simulink model "ScriptDemo"  (R2022b)
settings: configuration reference "TmVcThermal_Configuration_sub" (kept outside this file)
undefined symbols (not defined in the file or in its folder): aaaa, bbbb, cTmComprCtrl_D_u8HvacFlowTable_db, cTmComprCtrl_D_u8HvacFlowTable_sw, cTmComprCtrl_n_i16ChillCmpIMax, cTmComprCtrl_n_i16ChillCmpIMin, cTmComprCtrl_n_i16ChillCmpIMin666, cTmComprCtrl_n_i16ChillCmpPMax, cTmComprCtrl_n_i16ChillCmpPMin, cTmComprCtrl_n_i16CmpChillCoolRpmKiMax, cTmComprCtrl_n_i16CmpChillCoolRpmKiMin, cTmComprCtrl_n_i16CmpChillCoolRpmKpMax, cTmComprCtrl_n_i16CmpChillCoolRpmKpMin, cTmComprCtrl_n_i16CmpCoolRpmKiMax, cTmComprCtrl_n_i16CmpCoolRpmKiMin, cTmComprCtrl_n_i16CmpCoolRpmKpMax, cTmComprCtrl_n_i16CmpCoolRpmKpMin, cTmComprCtrl_n_i16SM4CmpHeatKiMax, cTmComprCtrl_n_i16SM4CmpHeatKiMin, cTmComprCtrl_n_i16SM4CmpHeatKpMax, cTmComprCtrl_n_i16SM4CmpHeatKpMin, cTmComprCtrl_n_i16SM5CmpHeatKiMax, cTmComprCtrl_n_i16SM5CmpHeatKiMin, cTmComprCtrl_n_i16SM5CmpHeatKpMax, cTmComprCtrl_n_i16SM5CmpHeatKpMin, cTmComprCtrl_n_i16SM6CmpHeatKiMax, cTmComprCtrl_n_i16SM6CmpHeatKiMin, cTmComprCtrl_n_i16SM6CmpHeatKpMax, cTmComprCtrl_n_i16SM6CmpHeatKpMin, cTmComprCtrl_n_u16CmpMaxSpdFanFltLimt, cTmComprCtrl_n_u16CmpMaxSpdLoSidePFltLimt, cTmComprCtrl_n_u16CmpMaxSpdSensorFltLimt, cTmComprCtrl_n_u16CompMinRpm, cTmComprCtrl_n_u16CompRpmIncThres, cTmComprCtrl_t_u16BattCooltFFPeriod, cTmComprCtrl_t_u16BattCooltPIPeriod, cTmComprCtrl_t_u16CmpCoolFFPeriod, cTmComprCtrl_t_u16CmpCoolPIPeriod, cTmComprCtrl_t_u16CoolCmpChillFFPeriod, cTmComprCtrl_t_u16CoolCmpChillPIPeriod, cTmComprCtrl_t_u16SM4CmpHeatFFPeriod, cTmComprCtrl_t_u16SM4CmpHeatPIPeriod, cTmComprCtrl_t_u16SM5CmpHeatFFPeriod, cTmComprCtrl_t_u16SM5CmpHeatPIPeriod, cTmComprCtrl_t_u16SM6CmpHeatFFPeriod, cTmComprCtrl_t_u16SM6CmpHeatPIPeriod, cTmComprCtrl_Te_EvapClearInteg, cTmComprCtrl_Te_i16HpReqTempSaturoffset, cTmComprCtrl_Te_i16SatLpReplaceDiff, cTmComprCtrl_Te_i16SM3BatDiffStartEvapDecOffset, cTmComprCtrl_Te_i16SM3EvapLo, cTmComprCtrl_Te_i16SM3TBatDiffEntEvapDecOffset, cTmComprCtrl_Te_i16SM3TBatDiffEntEvapDecOffsetQuit, cTmComprCtrl_Te_s32ErrCmpChillPIContinueCoolH, cTmComprCtrl_Te_s32ErrCmpChillPIContinueCoolL, cTmComprCtrl_Te_s32ErrCmpPIContinueChillH, cTmComprCtrl_Te_s32ErrCmpPIContinueChillL, cTmComprCtrl_Te_s32ErrCmpPIContinueCoolH, cTmComprCtrl_Te_s32ErrCmpPIContinueCoolL, cTmComprCtrl_Te_s32ErrCmpPIContinueHeatH ... (+398)
libraries: simulink x846, PCMULib x711, simulink_need_slupdate x4
(part 17 of 49)

== system ScriptDemo/Create/Model/createMode/Before ==
  note: % 目的: 为输出端口创建debug 及对应的输入模块
      | [cnt] = createDebug(gcs)
  sTmRefriVlvCtrl_X_s32CEXVPosReqIn : Inport  OutDataTypeStr=single
  sTmRefriVlvCtrl_X_s32EEXVPosReqIn : Inport  Port=2  OutDataTypeStr=single
  sTmRefriVlvCtrl_X_s32BEXVPosReqIn : Inport  Port=3  OutDataTypeStr=single
  yTmRefriVlvCtrl_B_HpcCexvMovEnableIn : Inport  Port=4  OutDataTypeStr=boolean
  sTmRefriVlvCtrl_Z_u8CEXVInitStateIn : Inport  Port=5  OutDataTypeStr=uint8
  yTmRefriVlvCtrl_B_CexvCalibReqIn : Inport  Port=6  OutDataTypeStr=boolean
  yTmRefriVlvCtrl_B_HpcEexvMovEnableIn : Inport  Port=7  OutDataTypeStr=boolean
  sTmRefriVlvCtrl_Z_u8EEXVInitStateIn : Inport  Port=8  OutDataTypeStr=uint8
  yTmRefriVlvCtrl_B_EexvCalibReqIn : Inport  Port=9  OutDataTypeStr=boolean
  yTmRefriVlvCtrl_B_HpcBexvMovEnableIn : Inport  Port=10  OutDataTypeStr=boolean
  sTmRefriVlvCtrl_Z_u8BEXVInitStateIn : Inport  Port=11  OutDataTypeStr=uint8
  yTmRefriVlvCtrl_B_BexvCalibReqIn : Inport  Port=12  OutDataTypeStr=boolean
  sTmRefriVlvCtrl_X_s32SM3BexvMaxPosIn : Inport  Port=13  OutDataTypeStr=single
  yTmRefriVlvCtrl_B_EvapBattTLimBexvEnaIn : Inport  Port=14  OutDataTypeStr=boolean
  sTmRefriVlvCtrl_D_u8EexvRefriSwitchStIn : Inport  Port=15  OutDataTypeStr=uint8
  sTmRefriVlvCtrl_D_u8CexvRefriSwitchStIn : Inport  Port=16  OutDataTypeStr=uint8
  sTmRefriVlvCtrl_D_u8BexvRefriSwitchStIn : Inport  Port=17  OutDataTypeStr=uint8
  OutDebug : PCMULib/Interface/OutdebugRvs  SWI=cTmRefriVlvCtrl_X_s32CEXVPosReq_sw  DBI=cTmRefriVlvCtrl_X_s32CEXVPosReq_db
      settings: SourceProductName=PCMULib
  OutDebug1 : PCMULib/Interface/OutdebugRvs  SWI=cTmRefriVlvCtrl_X_s32EEXVPosReq_sw  DBI=cTmRefriVlvCtrl_X_s32EEXVPosReq_db
      settings: SourceProductName=PCMULib
  OutDebug10 : PCMULib/Interface/OutdebugRvs  SWI=cTmRefriVlvCtrl_Z_u8BEXVInitState_sw  DBI=cTmRefriVlvCtrl_Z_u8BEXVInitState_db
      settings: SourceProductName=PCMULib
  OutDebug11 : PCMULib/Interface/OutdebugRvs  SWI=cTmRefriVlvCtrl_B_BexvCalibReq_sw  DBI=cTmRefriVlvCtrl_B_BexvCalibReq_db
      settings: SourceProductName=PCMULib
  OutDebug12 : PCMULib/Interface/OutdebugRvs  SWI=cTmRefriVlvCtrl_X_s32SM3BexvMaxPos_sw  DBI=cTmRefriVlvCtrl_X_s32SM3BexvMaxPos_db
      settings: SourceProductName=PCMULib
  OutDebug13 : PCMULib/Interface/OutdebugRvs  SWI=cTmRefriVlvCtrl_B_EvapBattTLimBexvEna_sw  DBI=cTmRefriVlvCtrl_B_EvapBattTLimBexvEna_db
      settings: SourceProductName=PCMULib
  OutDebug14 : PCMULib/Interface/OutdebugRvs  SWI=cTmRefriVlvCtrl_D_u8EexvRefriSwitchSt_sw  DBI=cTmRefriVlvCtrl_D_u8EexvRefriSwitchSt_db
      settings: SourceProductName=PCMULib
  OutDebug15 : PCMULib/Interface/OutdebugRvs  SWI=cTmRefriVlvCtrl_D_u8CexvRefriSwitchSt_sw  DBI=cTmRefriVlvCtrl_D_u8CexvRefriSwitchSt_db
      settings: SourceProductName=PCMULib
  OutDebug16 : PCMULib/Interface/OutdebugRvs  SWI=cTmRefriVlvCtrl_D_u8BexvRefriSwitchSt_sw  DBI=cTmRefriVlvCtrl_D_u8BexvRefriSwitchSt_db
      settings: SourceProductName=PCMULib
  OutDebug2 : PCMULib/Interface/OutdebugRvs  SWI=cTmRefriVlvCtrl_X_s32BEXVPosReq_sw  DBI=cTmRefriVlvCtrl_X_s32BEXVPosReq_db
      settings: SourceProductName=PCMULib
  OutDebug3 : PCMULib/Interface/OutdebugRvs  SWI=cTmRefriVlvCtrl_B_HpcCexvMovEnable_sw  DBI=cTmRefriVlvCtrl_B_HpcCexvMovEnable_db
      settings: SourceProductName=PCMULib
  OutDebug4 : PCMULib/Interface/OutdebugRvs  SWI=cTmRefriVlvCtrl_Z_u8CEXVInitState_sw  DBI=cTmRefriVlvCtrl_Z_u8CEXVInitState_db
      settings: SourceProductName=PCMULib
  OutDebug5 : PCMULib/Interface/OutdebugRvs  SWI=cTmRefriVlvCtrl_B_CexvCalibReq_sw  DBI=cTmRefriVlvCtrl_B_CexvCalibReq_db
      settings: SourceProductName=PCMULib
  OutDebug6 : PCMULib/Interface/OutdebugRvs  SWI=cTmRefriVlvCtrl_B_HpcEexvMovEnable_sw  DBI=cTmRefriVlvCtrl_B_HpcEexvMovEnable_db
      settings: SourceProductName=PCMULib
  OutDebug7 : PCMULib/Interface/OutdebugRvs  SWI=cTmRefriVlvCtrl_Z_u8EEXVInitState_sw  DBI=cTmRefriVlvCtrl_Z_u8EEXVInitState_db
      settings: SourceProductName=PCMULib
  OutDebug8 : PCMULib/Interface/OutdebugRvs  SWI=cTmRefriVlvCtrl_B_EexvCalibReq_sw  DBI=cTmRefriVlvCtrl_B_EexvCalibReq_db
      settings: SourceProductName=PCMULib
  OutDebug9 : PCMULib/Interface/OutdebugRvs  SWI=cTmRefriVlvCtrl_B_HpcBexvMovEnable_sw  DBI=cTmRefriVlvCtrl_B_HpcBexvMovEnable_db
      settings: SourceProductName=PCMULib
  sTmRefriVlvCtrl_X_s32CEXVPosReq : Outport  OutDataTypeStr=single
  sTmRefriVlvCtrl_X_s32EEXVPosReq : Outport  Port=2  OutDataTypeStr=single
  sTmRefriVlvCtrl_X_s32BEXVPosReq : Outport  Port=3  OutDataTypeStr=single
  yTmRefriVlvCtrl_B_HpcCexvMovEnable : Outport  Port=4  OutDataTypeStr=boolean
  sTmRefriVlvCtrl_Z_u8CEXVInitState : Outport  Port=5  OutDataTypeStr=uint8
  yTmRefriVlvCtrl_B_CexvCalibReq : Outport  Port=6  OutDataTypeStr=boolean
  yTmRefriVlvCtrl_B_HpcEexvMovEnable : Outport  Port=7  OutDataTypeStr=boolean
  sTmRefriVlvCtrl_Z_u8EEXVInitState : Outport  Port=8  OutDataTypeStr=uint8
  yTmRefriVlvCtrl_B_EexvCalibReq : Outport  Port=9  OutDataTypeStr=boolean
  yTmRefriVlvCtrl_B_HpcBexvMovEnable : Outport  Port=10  OutDataTypeStr=boolean
  sTmRefriVlvCtrl_Z_u8BEXVInitState : Outport  Port=11  OutDataTypeStr=uint8
  yTmRefriVlvCtrl_B_BexvCalibReq : Outport  Port=12  OutDataTypeStr=boolean
  sTmRefriVlvCtrl_X_s32SM3BexvMaxPos : Outport  Port=13  OutDataTypeStr=single
  yTmRefriVlvCtrl_B_EvapBattTLimBexvEna : Outport  Port=14  OutDataTypeStr=boolean
  sTmRefriVlvCtrl_D_u8EexvRefriSwitchSt : Outport  Port=15  OutDataTypeStr=uint8
  sTmRefriVlvCtrl_D_u8CexvRefriSwitchSt : Outport  Port=16  OutDataTypeStr=uint8
  sTmRefriVlvCtrl_D_u8BexvRefriSwitchSt : Outport  Port=17  OutDataTypeStr=uint8
  wires:
  sTmRefriVlvCtrl_X_s32SM3BexvMaxPosIn/1 -> OutDebug12/1
  OutDebug12/1 -> sTmRefriVlvCtrl_X_s32SM3BexvMaxPos/1
  sTmRefriVlvCtrl_X_s32BEXVPosReqIn/1 -> OutDebug2/1
  OutDebug2/1 -> sTmRefriVlvCtrl_X_s32BEXVPosReq/1
  OutDebug16/1 -> sTmRefriVlvCtrl_D_u8BexvRefriSwitchSt/1
  sTmRefriVlvCtrl_D_u8EexvRefriSwitchStIn/1 -> OutDebug14/1
  OutDebug5/1 -> yTmRefriVlvCtrl_B_CexvCalibReq/1
  OutDebug3/1 -> yTmRefriVlvCtrl_B_HpcCexvMovEnable/1
  sTmRefriVlvCtrl_Z_u8CEXVInitStateIn/1 -> OutDebug4/1
  OutDebug4/1 -> sTmRefriVlvCtrl_Z_u8CEXVInitState/1
  sTmRefriVlvCtrl_D_u8BexvRefriSwitchStIn/1 -> OutDebug16/1
  OutDebug1/1 -> sTmRefriVlvCtrl_X_s32EEXVPosReq/1
  OutDebug14/1 -> sTmRefriVlvCtrl_D_u8EexvRefriSwitchSt/1
  yTmRefriVlvCtrl_B_CexvCalibReqIn/1 -> OutDebug5/1
  sTmRefriVlvCtrl_X_s32EEXVPosReqIn/1 -> OutDebug1/1
  yTmRefriVlvCtrl_B_HpcCexvMovEnableIn/1 -> OutDebug3/1
  yTmRefriVlvCtrl_B_EvapBattTLimBexvEnaIn/1 -> OutDebug13/1
  OutDebug13/1 -> yTmRefriVlvCtrl_B_EvapBattTLimBexvEna/1
  sTmRefriVlvCtrl_Z_u8BEXVInitStateIn/1 -> OutDebug10/1
  OutDebug10/1 -> sTmRefriVlvCtrl_Z_u8BEXVInitState/1
  sTmRefriVlvCtrl_D_u8CexvRefriSwitchStIn/1 -> OutDebug15/1
  OutDebug15/1 -> sTmRefriVlvCtrl_D_u8CexvRefriSwitchSt/1
  OutDebug/1 -> sTmRefriVlvCtrl_X_s32CEXVPosReq/1
  OutDebug7/1 -> sTmRefriVlvCtrl_Z_u8EEXVInitState/1
  OutDebug8/1 -> yTmRefriVlvCtrl_B_EexvCalibReq/1
  yTmRefriVlvCtrl_B_EexvCalibReqIn/1 -> OutDebug8/1
  sTmRefriVlvCtrl_X_s32CEXVPosReqIn/1 -> OutDebug/1
  OutDebug6/1 -> yTmRefriVlvCtrl_B_HpcEexvMovEnable/1
  yTmRefriVlvCtrl_B_HpcEexvMovEnableIn/1 -> OutDebug6/1
  sTmRefriVlvCtrl_Z_u8EEXVInitStateIn/1 -> OutDebug7/1
  yTmRefriVlvCtrl_B_HpcBexvMovEnableIn/1 -> OutDebug9/1
  OutDebug9/1 -> yTmRefriVlvCtrl_B_HpcBexvMovEnable/1
  yTmRefriVlvCtrl_B_BexvCalibReqIn/1 -> OutDebug11/1
  OutDebug11/1 -> yTmRefriVlvCtrl_B_BexvCalibReq/1

== system ScriptDemo/Create/Model/createMode/Subsystem ==
  yTmIn_B_CPSRFbSt : Inport  OutDataTypeStr=boolean
  sTmIn_D_u8CexvCalibSts : Inport  Port=2  OutDataTypeStr=uint8
  sTmDiag_D_u8EexvFltSt : Inport  Port=3  OutDataTypeStr=uint8
  sTmDiag_D_u8CexvFltSt : Inport  Port=4  OutDataTypeStr=uint8
  sTmRefriVlvCtrl_X_s32CEXVPosReq : Outport  OutDataTypeStr=single
  sTmRefriVlvCtrl_X_s32EEXVPosReq : Outport  Port=2  OutDataTypeStr=single
  sTmRefriVlvCtrl_X_s32BEXVPosReq : Outport  Port=3  OutDataTypeStr=single
  yTmRefriVlvCtrl_B_HpcCexvMovEnable : Outport  Port=4  OutDataTypeStr=boolean
  sTmRefriVlvCtrl_Z_u8CEXVInitState : Outport  Port=5  OutDataTypeStr=uint8
  wires:
  yTmIn_B_CPSRFbSt/1 -> [yTmIn_B_CPSRFbSt]
  sTmIn_D_u8CexvCalibSts/1 -> [sTmIn_D_u8CexvCalibSts]
  ? -> [sTmIn_D_u8EexvCalibSts]
  ? -> [sTmIn_D_u8BexvCalibSts]
  ? -> [sTmDiag_D_u8BexvFltSt]
  sTmDiag_D_u8EexvFltSt/1 -> [sTmDiag_D_u8EexvFltSt]
  sTmDiag_D_u8CexvFltSt/1 -> [sTmDiag_D_u8CexvFltSt]
  [sTmRefriVlvCtrl_X_s32CEXVPosReq] -> sTmRefriVlvCtrl_X_s32CEXVPosReq/1
  [sTmRefriVlvCtrl_X_s32EEXVPosReq] -> sTmRefriVlvCtrl_X_s32EEXVPosReq/1
  [sTmRefriVlvCtrl_X_s32BEXVPosReq] -> sTmRefriVlvCtrl_X_s32BEXVPosReq/1
  [yTmRefriVlvCtrl_B_HpcCexvMovEnable] -> yTmRefriVlvCtrl_B_HpcCexvMovEnable/1
  [sTmRefriVlvCtrl_Z_u8CEXVInitState] -> sTmRefriVlvCtrl_Z_u8CEXVInitState/1

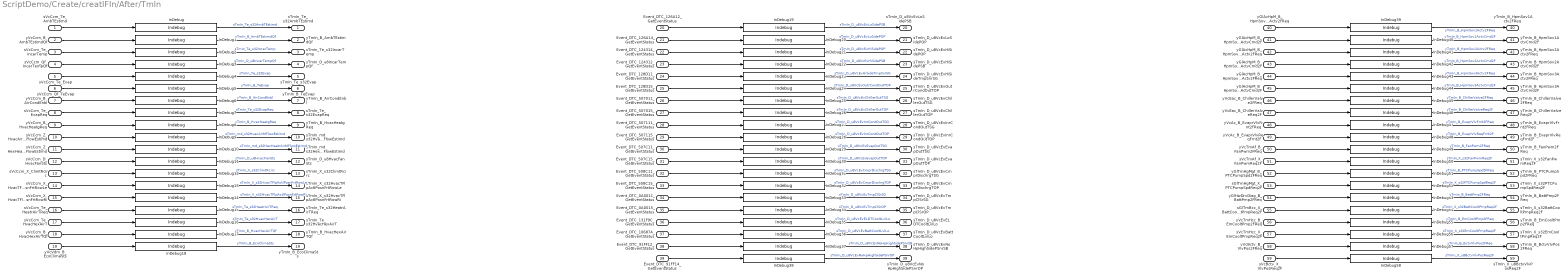
== system ScriptDemo/Create/creatIFIn/After/TmIn ==
  sVcCcm_Te_AmbTEstimd : Inport  OutDataTypeStr=single
  yVcCcm_B_AmbTEstimdQf : Inport  Port=2  OutDataTypeStr=boolean
  sVcCcm_Te_IncarTemp : Inport  Port=3  OutDataTypeStr=single
  sVcCcm_Qf_IncarTempQf : Inport  Port=4  OutDataTypeStr=uint8
  sVcCcm_Te_Evap : Inport  Port=5  OutDataTypeStr=single
  sVcCcm_Qf_TeEvap : Inport  Port=6  OutDataTypeStr=boolean
  yVcCcm_B_AirCondEnbl : Inport  Port=7  OutDataTypeStr=boolean
  sVcCcm_Te_EvapReq : Inport  Port=8  OutDataTypeStr=single
  yVcCcm_B_HvacHeatgReq : Inport  Port=9  OutDataTypeStr=boolean
  sVcCcm_Z_HvacAirMFlowEstimd : Inport  Port=10  OutDataTypeStr=single
  sVcCcm_Z_HexHeatrAirMFlowEstimd : Inport  Port=11  OutDataTypeStr=single
  sVcCcm_D_HvacFanSts : Inport  Port=12  OutDataTypeStr=uint8
  sVcCcm_X_ClimtRcirc : Inport  Port=13  OutDataTypeStr=single
  sVcCcm_X_HvacTFlpActlPosnFrtRowLe : Inport  Port=14  OutDataTypeStr=single
  sVcCcm_X_HvacTFlpActlPosnFrtRowRi : Inport  Port=15  OutDataTypeStr=single
  sVcCcm_Te_HeatrAirTReq : Inport  Port=16  OutDataTypeStr=single
  sVcCcm_Te_HvacHexAirT : Inport  Port=17  OutDataTypeStr=single
  yVcCcm_B_HvacHexAirTQf : Inport  Port=18  OutDataTypeStr=boolean
  yVcVdm_B_EcoClimaSts : Inport  Port=19  OutDataTypeStr=boolean
  Event_DTC_126A12_GetEventStatus : Inport  Port=20  OutDataTypeStr=uint8
  Event_DTC_126A14_GetEventStatus : Inport  Port=21  OutDataTypeStr=uint8
  Event_DTC_124314_GetEventStatus : Inport  Port=22  OutDataTypeStr=uint8
  Event_DTC_124312_GetEventStatus : Inport  Port=23  OutDataTypeStr=uint8
  Event_DTC_128D11_GetEventStatus : Inport  Port=24  OutDataTypeStr=uint8
  Event_DTC_128D15_GetEventStatus : Inport  Port=25  OutDataTypeStr=uint8
  Event_DTC_507011_GetEventStatus : Inport  Port=26  OutDataTypeStr=uint8
  Event_DTC_507015_GetEventStatus : Inport  Port=27  OutDataTypeStr=uint8
  Event_DTC_507111_GetEventStatus : Inport  Port=28  OutDataTypeStr=uint8
  Event_DTC_507115_GetEventStatus : Inport  Port=29  OutDataTypeStr=uint8
  Event_DTC_507C11_GetEventStatus : Inport  Port=30  OutDataTypeStr=uint8
  Event_DTC_507C15_GetEventStatus : Inport  Port=31  OutDataTypeStr=uint8
  Event_DTC_508C11_GetEventStatus : Inport  Port=32  OutDataTypeStr=uint8
  Event_DTC_508C15_GetEventStatus : Inport  Port=33  OutDataTypeStr=uint8
  Event_DTC_0A0011_GetEventStatus : Inport  Port=34  OutDataTypeStr=uint8
  Event_DTC_0A0015_GetEventStatus : Inport  Port=35  OutDataTypeStr=uint8
  Event_DTC_131F9C_GetEventStatus : Inport  Port=36  OutDataTypeStr=uint8
  Event_DTC_10687A_GetEventStatus : Inport  Port=37  OutDataTypeStr=uint8
  Event_DTC_91FF12_GetEventStatus : Inport  Port=38  OutDataTypeStr=uint8
  Event_DTC_91FF14_GetEventStatus : Inport  Port=39  OutDataTypeStr=uint8
  yGlAcHpM_B_HpmSov1Actv2FReq : Inport  Port=40  OutDataTypeStr=boolean
  yGlAcHpM_B_HpmSov1ActvCmd2F : Inport  Port=41  OutDataTypeStr=boolean
  yGlAcHpM_B_HpmSov2Actv2FReq : Inport  Port=42  OutDataTypeStr=boolean
  yGlAcHpM_B_HpmSov2ActvCmd2F : Inport  Port=43  OutDataTypeStr=boolean
  yGlAcHpM_B_HpmSov3Actv2FReq : Inport  Port=44  OutDataTypeStr=boolean
  yGlAcHpM_B_HpmSov3ActvCmd2F : Inport  Port=45  OutDataTypeStr=boolean
  yVcEac_B_ChillerValve2FReq : Inport  Port=46  OutDataTypeStr=boolean
  yVcEac_B_ChillerValveReq2F : Inport  Port=47  OutDataTypeStr=boolean
  yVcAc_B_EvaprVlvFrnt2FReq : Inport  Port=48  OutDataTypeStr=boolean
  yVcAc_B_EvaprVlvReqFrnt2F : Inport  Port=49  OutDataTypeStr=boolean
  yVcTmAf_B_FanPwm2FReq : Inport  Port=50  OutDataTypeStr=boolean
  sVcTmAf_X_FanPwmReq2F : Inport  Port=51  OutDataTypeStr=single
  yGlTmHgMgt_B_PTCPumpSpd2FReq : Inport  Port=52  OutDataTypeStr=boolean
  sGlTmHgMgt_X_PTCPumpSpdReq2F : Inport  Port=53  OutDataTypeStr=single
  yGlHwDrvDiag_B_BattPmp2FReq : Inport  Port=54  OutDataTypeStr=boolean
  sGlTmBcc_X_BattCooltPmpReq2F : Inport  Port=55  OutDataTypeStr=single
  yVcTmHcc_B_EmCooltPmp2FReq : Inport  Port=56  OutDataTypeStr=boolean
  sVcTmHcc_X_EmCooltPmpReq2F : Inport  Port=57  OutDataTypeStr=single
  yVcBctv_B_VlvPos2FReq : Inport  Port=58  OutDataTypeStr=boolean
  sVcBctv_X_VlvPosReq2F : Inport  Port=59  OutDataTypeStr=uint8
  InDebug : PCMULib/Interface/Indebug  SWI=cTmIn_Te_s32AmbTEstimd_swi  DBI=cTmIn_Te_s32AmbTEstimd_dbi
      settings: SourceProductName=PCMULib
  InDebug1 : PCMULib/Interface/Indebug  SWI=cTmIn_B_AmbTEstimdQf_swi  DBI=cTmIn_B_AmbTEstimdQf_dbi
      settings: SourceProductName=PCMULib
  InDebug10 : PCMULib/Interface/Indebug  SWI=cTmIn_md_s32HexHeatrAirMFlowEstimd_swi  DBI=cTmIn_md_s32HexHeatrAirMFlowEstimd_dbi
      settings: SourceProductName=PCMULib
  InDebug11 : PCMULib/Interface/Indebug  SWI=cTmIn_D_u8HvacFanSts_swi  DBI=cTmIn_D_u8HvacFanSts_dbi
      settings: SourceProductName=PCMULib
  InDebug12 : PCMULib/Interface/Indebug  SWI=cTmIn_X_s32ClimtRcirc_swi  DBI=cTmIn_X_s32ClimtRcirc_dbi
      settings: SourceProductName=PCMULib
  InDebug13 : PCMULib/Interface/Indebug  SWI=cTmIn_X_s32HvacTFlpActlPosnFrtRowLe_swi  DBI=cTmIn_X_s32HvacTFlpActlPosnFrtRowLe_dbi
      settings: SourceProductName=PCMULib
  InDebug14 : PCMULib/Interface/Indebug  SWI=cTmIn_X_s32HvacTFlpActlPosnFrtRowRi_swi  DBI=cTmIn_X_s32HvacTFlpActlPosnFrtRowRi_dbi
      settings: SourceProductName=PCMULib
  InDebug15 : PCMULib/Interface/Indebug  SWI=cTmIn_Te_s32HeatrAirTReq_swi  DBI=cTmIn_Te_s32HeatrAirTReq_dbi
      settings: SourceProductName=PCMULib
  InDebug16 : PCMULib/Interface/Indebug  SWI=cTmIn_Te_s32HvacHexAirT_swi  DBI=cTmIn_Te_s32HvacHexAirT_dbi
      settings: SourceProductName=PCMULib
  InDebug17 : PCMULib/Interface/Indebug  SWI=cTmIn_B_HvacHexAirTQf_swi  DBI=cTmIn_B_HvacHexAirTQf_dbi
      settings: SourceProductName=PCMULib
  InDebug18 : PCMULib/Interface/Indebug  SWI=cTmIn_B_EcoClimaSts_swi  DBI=cTmIn_B_EcoClimaSts_dbi
      settings: SourceProductName=PCMULib
  InDebug19 : PCMULib/Interface/Indebug  SWI=cTmIn_D_u8VcEvLoSidePSB_swi  DBI=cTmIn_D_u8VcEvLoSidePSB_dbi
      settings: SourceProductName=PCMULib
  InDebug2 : PCMULib/Interface/Indebug  SWI=cTmIn_Te_s32IncarTemp_swi  DBI=cTmIn_Te_s32IncarTemp_dbi
      settings: SourceProductName=PCMULib
  InDebug20 : PCMULib/Interface/Indebug  SWI=cTmIn_D_u8VcEvLoSidePOP_swi  DBI=cTmIn_D_u8VcEvLoSidePOP_dbi
      settings: SourceProductName=PCMULib
  InDebug21 : PCMULib/Interface/Indebug  SWI=cTmIn_D_u8VcEvHiSidePOP_swi  DBI=cTmIn_D_u8VcEvHiSidePOP_dbi
      settings: SourceProductName=PCMULib
  InDebug22 : PCMULib/Interface/Indebug  SWI=cTmIn_D_u8VcEvHiSidePSB_swi  DBI=cTmIn_D_u8VcEvHiSidePSB_dbi
      settings: SourceProductName=PCMULib
  InDebug23 : PCMULib/Interface/Indebug  SWI=cTmIn_D_u8VcEvHiSideTmpSnrSG_swi  DBI=cTmIn_D_u8VcEvHiSideTmpSnrSG_dbi
      settings: SourceProductName=PCMULib
  InDebug24 : PCMULib/Interface/Indebug  SWI=cTmIn_D_u8VcEvOutrCondOutTOP_swi  DBI=cTmIn_D_u8VcEvOutrCondOutTOP_dbi
      settings: SourceProductName=PCMULib
  InDebug25 : PCMULib/Interface/Indebug  SWI=cTmIn_D_u8VcEvChillerOutTSG_swi  DBI=cTmIn_D_u8VcEvChillerOutTSG_dbi
      settings: SourceProductName=PCMULib
  InDebug26 : PCMULib/Interface/Indebug  SWI=cTmIn_D_u8VcEvChillerOutTOP_swi  DBI=cTmIn_D_u8VcEvChillerOutTOP_dbi
      settings: SourceProductName=PCMULib
  InDebug27 : PCMULib/Interface/Indebug  SWI=cTmIn_D_u8VcEvInrCondOutTSG_swi  DBI=cTmIn_D_u8VcEvInrCondOutTSG_dbi
      settings: SourceProductName=PCMULib
  InDebug28 : PCMULib/Interface/Indebug  SWI=cTmIn_D_u8VcEvInrCondOutTOP_swi  DBI=cTmIn_D_u8VcEvInrCondOutTOP_dbi
      settings: SourceProductName=PCMULib
  InDebug29 : PCMULib/Interface/Indebug  SWI=cTmIn_D_u8VcEvEvapOutTSG_swi  DBI=cTmIn_D_u8VcEvEvapOutTSG_dbi
      settings: SourceProductName=PCMULib
  InDebug3 : PCMULib/Interface/Indebug  SWI=cTmIn_D_u8IncarTempQf_swi  DBI=cTmIn_D_u8IncarTempQf_dbi
      settings: SourceProductName=PCMULib
  InDebug30 : PCMULib/Interface/Indebug  SWI=cTmIn_D_u8VcEvEvapOutTOP_swi  DBI=cTmIn_D_u8VcEvEvapOutTOP_dbi
      settings: SourceProductName=PCMULib
  InDebug31 : PCMULib/Interface/Indebug  SWI=cTmIn_D_u8VcEvCmprDischrgTSG_swi  DBI=cTmIn_D_u8VcEvCmprDischrgTSG_dbi
      settings: SourceProductName=PCMULib
  InDebug32 : PCMULib/Interface/Indebug  SWI=cTmIn_D_u8VcEvCmprDischrgTOP_swi  DBI=cTmIn_D_u8VcEvCmprDischrgTOP_dbi
      settings: SourceProductName=PCMULib
  InDebug33 : PCMULib/Interface/Indebug  SWI=cTmIn_D_u8VcEvTmpClSrSG_swi  DBI=cTmIn_D_u8VcEvTmpClSrSG_dbi
      settings: SourceProductName=PCMULib
  InDebug34 : PCMULib/Interface/Indebug  SWI=cTmIn_D_u8VcEvTmpClSrOP_swi  DBI=cTmIn_D_u8VcEvTmpClSrOP_dbi
      settings: SourceProductName=PCMULib
  InDebug35 : PCMULib/Interface/Indebug  SWI=cTmIn_D_u8VcEvELDTCooltLvlLo_swi  DBI=cTmIn_D_u8VcEvELDTCooltLvlLo_dbi
      settings: SourceProductName=PCMULib
  InDebug36 : PCMULib/Interface/Indebug  SWI=cTmIn_D_u8VcEvBattCooltLvlLo_swi  DBI=cTmIn_D_u8VcEvBattCooltLvlLo_dbi
      settings: SourceProductName=PCMULib
  InDebug37 : PCMULib/Interface/Indebug  SWI=cTmIn_D_u8VcEvNoHpHighSidePSnrSB_swi  DBI=cTmIn_D_u8VcEvNoHpHighSidePSnrSB_dbi
      settings: SourceProductName=PCMULib
  InDebug38 : PCMULib/Interface/Indebug  SWI=cTmIn_D_u8VcEvNoHpHighSidePSnrOP_swi  DBI=cTmIn_D_u8VcEvNoHpHighSidePSnrOP_dbi
      settings: SourceProductName=PCMULib
  InDebug39 : PCMULib/Interface/Indebug  SWI=cTmIn_B_HpmSov1Actv2FReq_swi  DBI=cTmIn_B_HpmSov1Actv2FReq_dbi
      settings: SourceProductName=PCMULib
  InDebug4 : PCMULib/Interface/Indebug  SWI=cTmIn_Te_s32Evap_swi  DBI=cTmIn_Te_s32Evap_dbi
      settings: SourceProductName=PCMULib
  InDebug40 : PCMULib/Interface/Indebug  SWI=cTmIn_B_HpmSov1ActvCmd2F_swi  DBI=cTmIn_B_HpmSov1ActvCmd2F_dbi
      settings: SourceProductName=PCMULib
  InDebug41 : PCMULib/Interface/Indebug  SWI=cTmIn_B_HpmSov2Actv2FReq_swi  DBI=cTmIn_B_HpmSov2Actv2FReq_dbi
      settings: SourceProductName=PCMULib
  InDebug42 : PCMULib/Interface/Indebug  SWI=cTmIn_B_HpmSov2ActvCmd2F_swi  DBI=cTmIn_B_HpmSov2ActvCmd2F_dbi
      settings: SourceProductName=PCMULib
  InDebug43 : PCMULib/Interface/Indebug  SWI=cTmIn_B_HpmSov3Actv2FReq_swi  DBI=cTmIn_B_HpmSov3Actv2FReq_dbi
      settings: SourceProductName=PCMULib
  InDebug44 : PCMULib/Interface/Indebug  SWI=cTmIn_B_HpmSov3ActvCmd2F_swi  DBI=cTmIn_B_HpmSov3ActvCmd2F_dbi
      settings: SourceProductName=PCMULib
  InDebug45 : PCMULib/Interface/Indebug  SWI=cTmIn_B_ChillerValve2FReq_swi  DBI=cTmIn_B_ChillerValve2FReq_dbi
      settings: SourceProductName=PCMULib
  InDebug46 : PCMULib/Interface/Indebug  SWI=cTmIn_B_ChillerValveReq2F_swi  DBI=cTmIn_B_ChillerValveReq2F_dbi
      settings: SourceProductName=PCMULib
  InDebug47 : PCMULib/Interface/Indebug  SWI=cTmIn_B_EvaprVlvFrnt2FReq_swi  DBI=cTmIn_B_EvaprVlvFrnt2FReq_dbi
      settings: SourceProductName=PCMULib
  InDebug48 : PCMULib/Interface/Indebug  SWI=cTmIn_B_EvaprVlvReqFrnt2F_swi  DBI=cTmIn_B_EvaprVlvReqFrnt2F_dbi
      settings: SourceProductName=PCMULib
  InDebug49 : PCMULib/Interface/Indebug  SWI=cTmIn_B_FanPwm2FReq_swi  DBI=cTmIn_B_FanPwm2FReq_dbi
      settings: SourceProductName=PCMULib
  InDebug5 : PCMULib/Interface/Indebug  SWI=cTmIn_B_TeEvap_swi  DBI=cTmIn_B_TeEvap_dbi
      settings: SourceProductName=PCMULib
  InDebug50 : PCMULib/Interface/Indebug  SWI=cTmIn_X_s32FanPwmReq2F_swi  DBI=cTmIn_X_s32FanPwmReq2F_dbi
      settings: SourceProductName=PCMULib
  InDebug51 : PCMULib/Interface/Indebug  SWI=cTmIn_B_PTCPumpSpd2FReq_swi  DBI=cTmIn_B_PTCPumpSpd2FReq_dbi
      settings: SourceProductName=PCMULib
  InDebug52 : PCMULib/Interface/Indebug  SWI=cTmIn_X_s32PTCPumpSpdReq2F_swi  DBI=cTmIn_X_s32PTCPumpSpdReq2F_dbi
      settings: SourceProductName=PCMULib
  InDebug53 : PCMULib/Interface/Indebug  SWI=cTmIn_B_BattPmp2FReq_swi  DBI=cTmIn_B_BattPmp2FReq_dbi
      settings: SourceProductName=PCMULib
  InDebug54 : PCMULib/Interface/Indebug  SWI=cTmIn_X_s32BattCooltPmpReq2F_swi  DBI=cTmIn_X_s32BattCooltPmpReq2F_dbi
      settings: SourceProductName=PCMULib
  InDebug55 : PCMULib/Interface/Indebug  SWI=cTmIn_B_EmCooltPmp2FReq_swi  DBI=cTmIn_B_EmCooltPmp2FReq_dbi
      settings: SourceProductName=PCMULib
  InDebug56 : PCMULib/Interface/Indebug  SWI=cTmIn_X_s32EmCooltPmpReq2F_swi  DBI=cTmIn_X_s32EmCooltPmpReq2F_dbi
      settings: SourceProductName=PCMULib
  InDebug57 : PCMULib/Interface/Indebug  SWI=cTmIn_B_BctvVlvPos2FReq_swi  DBI=cTmIn_B_BctvVlvPos2FReq_dbi
      settings: SourceProductName=PCMULib
  InDebug58 : PCMULib/Interface/Indebug  SWI=cTmIn_X_u8BctvVlvPosReq2F_swi  DBI=cTmIn_X_u8BctvVlvPosReq2F_dbi
      settings: SourceProductName=PCMULib
  InDebug6 : PCMULib/Interface/Indebug  SWI=cTmIn_B_AirCondEnbl_swi  DBI=cTmIn_B_AirCondEnbl_dbi
      settings: SourceProductName=PCMULib
  InDebug7 : PCMULib/Interface/Indebug  SWI=cTmIn_Te_s32EvapReq_swi  DBI=cTmIn_Te_s32EvapReq_dbi
      settings: SourceProductName=PCMULib
  InDebug8 : PCMULib/Interface/Indebug  SWI=cTmIn_B_HvacHeatgReq_swi  DBI=cTmIn_B_HvacHeatgReq_dbi
      settings: SourceProductName=PCMULib
  InDebug9 : PCMULib/Interface/Indebug  SWI=cTmIn_md_s32HvacAirMFlowEstimd_swi  DBI=cTmIn_md_s32HvacAirMFlowEstimd_dbi
      settings: SourceProductName=PCMULib
  sTmIn_Te_s32AmbTEstimd : Outport  OutDataTypeStr=single
  yTmIn_B_AmbTEstimdQf : Outport  Port=2  OutDataTypeStr=boolean
  sTmIn_Te_s32IncarTemp : Outport  Port=3  OutDataTypeStr=single
  sTmIn_D_u8IncarTempQf : Outport  Port=4  OutDataTypeStr=uint8
  sTmIn_Te_s32Evap : Outport  Port=5  OutDataTypeStr=single
  yTmIn_B_TeEvap : Outport  Port=6  OutDataTypeStr=boolean
  yTmIn_B_AirCondEnbl : Outport  Port=7  OutDataTypeStr=boolean
  sTmIn_Te_s32EvapReq : Outport  Port=8  OutDataTypeStr=single
  yTmIn_B_HvacHeatgReq : Outport  Port=9  OutDataTypeStr=boolean
  sTmIn_md_s32HvacAirMFlowEstimd : Outport  Port=10  OutDataTypeStr=single
  sTmIn_md_s32HexHeatrAirMFlowEstimd : Outport  Port=11  OutDataTypeStr=single
  sTmIn_D_u8HvacFanSts : Outport  Port=12  OutDataTypeStr=uint8
  sTmIn_X_s32ClimtRcirc : Outport  Port=13  OutDataTypeStr=single
  sTmIn_X_s32HvacTFlpActlPosnFrtRowLe : Outport  Port=14  OutDataTypeStr=single
  sTmIn_X_s32HvacTFlpActlPosnFrtRowRi : Outport  Port=15  OutDataTypeStr=single
  sTmIn_Te_s32HeatrAirTReq : Outport  Port=16  OutDataTypeStr=single
  sTmIn_Te_s32HvacHexAirT : Outport  Port=17  OutDataTypeStr=single
  yTmIn_B_HvacHexAirTQf : Outport  Port=18  OutDataTypeStr=boolean
  yTmIn_B_EcoClimaSts : Outport  Port=19  OutDataTypeStr=boolean
  sTmIn_D_u8VcEvLoSidePSB : Outport  Port=20  OutDataTypeStr=uint8
  sTmIn_D_u8VcEvLoSidePOP : Outport  Port=21  OutDataTypeStr=uint8
  sTmIn_D_u8VcEvHiSidePOP : Outport  Port=22  OutDataTypeStr=uint8
  sTmIn_D_u8VcEvHiSidePSB : Outport  Port=23  OutDataTypeStr=uint8
  sTmIn_D_u8VcEvHiSideTmpSnrSG : Outport  Port=24  OutDataTypeStr=uint8
  sTmIn_D_u8VcEvOutrCondOutTOP : Outport  Port=25  OutDataTypeStr=uint8
  sTmIn_D_u8VcEvChillerOutTSG : Outport  Port=26  OutDataTypeStr=uint8
  sTmIn_D_u8VcEvChillerOutTOP : Outport  Port=27  OutDataTypeStr=uint8
  sTmIn_D_u8VcEvInrCondOutTSG : Outport  Port=28  OutDataTypeStr=uint8
  sTmIn_D_u8VcEvInrCondOutTOP : Outport  Port=29  OutDataTypeStr=uint8
  sTmIn_D_u8VcEvEvapOutTSG : Outport  Port=30  OutDataTypeStr=uint8
  sTmIn_D_u8VcEvEvapOutTOP : Outport  Port=31  OutDataTypeStr=uint8
  sTmIn_D_u8VcEvCmprDischrgTSG : Outport  Port=32  OutDataTypeStr=uint8
  sTmIn_D_u8VcEvCmprDischrgTOP : Outport  Port=33  OutDataTypeStr=uint8
  sTmIn_D_u8VcEvTmpClSrSG : Outport  Port=34  OutDataTypeStr=uint8
  sTmIn_D_u8VcEvTmpClSrOP : Outport  Port=35  OutDataTypeStr=uint8
  sTmIn_D_u8VcEvELDTCooltLvlLo : Outport  Port=36  OutDataTypeStr=uint8
  sTmIn_D_u8VcEvBattCooltLvlLo : Outport  Port=37  OutDataTypeStr=uint8
  sTmIn_D_u8VcEvNoHpHighSidePSnrSB : Outport  Port=38  OutDataTypeStr=uint8
  sTmIn_D_u8VcEvNoHpHighSidePSnrOP : Outport  Port=39  OutDataTypeStr=uint8
  yTmIn_B_HpmSov1Actv2FReq : Outport  Port=40  OutDataTypeStr=boolean
  yTmIn_B_HpmSov1ActvCmd2F : Outport  Port=41  OutDataTypeStr=boolean
  yTmIn_B_HpmSov2Actv2FReq : Outport  Port=42  OutDataTypeStr=boolean
  yTmIn_B_HpmSov2ActvCmd2F : Outport  Port=43  OutDataTypeStr=boolean
  yTmIn_B_HpmSov3Actv2FReq : Outport  Port=44  OutDataTypeStr=boolean
  yTmIn_B_HpmSov3ActvCmd2F : Outport  Port=45  OutDataTypeStr=boolean
  yTmIn_B_ChillerValve2FReq : Outport  Port=46  OutDataTypeStr=boolean
  yTmIn_B_ChillerValveReq2F : Outport  Port=47  OutDataTypeStr=boolean
  yTmIn_B_EvaprVlvFrnt2FReq : Outport  Port=48  OutDataTypeStr=boolean
  yTmIn_B_EvaprVlvReqFrnt2F : Outport  Port=49  OutDataTypeStr=boolean
  yTmIn_B_FanPwm2FReq : Outport  Port=50  OutDataTypeStr=boolean
  sTmIn_X_s32FanPwmReq2F : Outport  Port=51  OutDataTypeStr=single
  yTmIn_B_PTCPumpSpd2FReq : Outport  Port=52  OutDataTypeStr=boolean
  sTmIn_X_s32PTCPumpSpdReq2F : Outport  Port=53  OutDataTypeStr=single
  yTmIn_B_BattPmp2FReq : Outport  Port=54  OutDataTypeStr=boolean
  sTmIn_X_s32BattCooltPmpReq2F : Outport  Port=55  OutDataTypeStr=single
  yTmIn_B_EmCooltPmp2FReq : Outport  Port=56  OutDataTypeStr=boolean
  sTmIn_X_s32EmCooltPmpReq2F : Outport  Port=57  OutDataTypeStr=single
  yTmIn_B_BctvVlvPos2FReq : Outport  Port=58  OutDataTypeStr=boolean
  sTmIn_X_u8BctvVlvPosReq2F : Outport  Port=59  OutDataTypeStr=uint8
  wires:
  sVcCcm_Te_AmbTEstimd/1 -> InDebug/1
  InDebug/1 -> sTmIn_Te_s32AmbTEstimd/1  "sTmIn_Te_s32AmbTEstimd"
  yVcCcm_B_AmbTEstimdQf/1 -> InDebug1/1
  InDebug1/1 -> yTmIn_B_AmbTEstimdQf/1  "yTmIn_B_AmbTEstimdQf"
  sVcCcm_Te_IncarTemp/1 -> InDebug2/1
  InDebug2/1 -> sTmIn_Te_s32IncarTemp/1  "sTmIn_Te_s32IncarTemp"
  sVcCcm_Qf_IncarTempQf/1 -> InDebug3/1
  InDebug3/1 -> sTmIn_D_u8IncarTempQf/1  "sTmIn_D_u8IncarTempQf"
  sVcCcm_Te_Evap/1 -> InDebug4/1
  InDebug4/1 -> sTmIn_Te_s32Evap/1  "sTmIn_Te_s32Evap"
  sVcCcm_Qf_TeEvap/1 -> InDebug5/1
  InDebug5/1 -> yTmIn_B_TeEvap/1  "yTmIn_B_TeEvap"
  yVcCcm_B_AirCondEnbl/1 -> InDebug6/1
  InDebug6/1 -> yTmIn_B_AirCondEnbl/1  "yTmIn_B_AirCondEnbl"
  sVcCcm_Te_EvapReq/1 -> InDebug7/1
  InDebug7/1 -> sTmIn_Te_s32EvapReq/1  "sTmIn_Te_s32EvapReq"
  yVcCcm_B_HvacHeatgReq/1 -> InDebug8/1
  InDebug8/1 -> yTmIn_B_HvacHeatgReq/1  "yTmIn_B_HvacHeatgReq"
  sVcCcm_Z_HvacAirMFlowEstimd/1 -> InDebug9/1
  InDebug9/1 -> sTmIn_md_s32HvacAirMFlowEstimd/1  "sTmIn_md_s32HvacAirMFlowEstimd"
  sVcCcm_Z_HexHeatrAirMFlowEstimd/1 -> InDebug10/1
  InDebug10/1 -> sTmIn_md_s32HexHeatrAirMFlowEstimd/1  "sTmIn_md_s32HexHeatrAirMFlowEstimd"
  sVcCcm_D_HvacFanSts/1 -> InDebug11/1
  InDebug11/1 -> sTmIn_D_u8HvacFanSts/1  "sTmIn_D_u8HvacFanSts"
  sVcCcm_X_ClimtRcirc/1 -> InDebug12/1
  InDebug12/1 -> sTmIn_X_s32ClimtRcirc/1  "sTmIn_X_s32ClimtRcirc"
  sVcCcm_X_HvacTFlpActlPosnFrtRowLe/1 -> InDebug13/1
  InDebug13/1 -> sTmIn_X_s32HvacTFlpActlPosnFrtRowLe/1  "sTmIn_X_s32HvacTFlpActlPosnFrtRowLe"
  sVcCcm_X_HvacTFlpActlPosnFrtRowRi/1 -> InDebug14/1
  InDebug14/1 -> sTmIn_X_s32HvacTFlpActlPosnFrtRowRi/1  "sTmIn_X_s32HvacTFlpActlPosnFrtRowRi"
  sVcCcm_Te_HeatrAirTReq/1 -> InDebug15/1
  InDebug15/1 -> sTmIn_Te_s32HeatrAirTReq/1  "sTmIn_Te_s32HeatrAirTReq"
  sVcCcm_Te_HvacHexAirT/1 -> InDebug16/1
  InDebug16/1 -> sTmIn_Te_s32HvacHexAirT/1  "sTmIn_Te_s32HvacHexAirT"
  yVcCcm_B_HvacHexAirTQf/1 -> InDebug17/1
  InDebug17/1 -> yTmIn_B_HvacHexAirTQf/1  "yTmIn_B_HvacHexAirTQf"
  yVcVdm_B_EcoClimaSts/1 -> InDebug18/1
  InDebug18/1 -> yTmIn_B_EcoClimaSts/1  "yTmIn_B_EcoClimaSts"
  Event_DTC_126A12_GetEventStatus/1 -> InDebug19/1
  InDebug19/1 -> sTmIn_D_u8VcEvLoSidePSB/1  "sTmIn_D_u8VcEvLoSidePSB"
  Event_DTC_126A14_GetEventStatus/1 -> InDebug20/1
  InDebug20/1 -> sTmIn_D_u8VcEvLoSidePOP/1  "sTmIn_D_u8VcEvLoSidePOP"
  Event_DTC_124314_GetEventStatus/1 -> InDebug21/1
  InDebug21/1 -> sTmIn_D_u8VcEvHiSidePOP/1  "sTmIn_D_u8VcEvHiSidePOP"
  Event_DTC_124312_GetEventStatus/1 -> InDebug22/1
  InDebug22/1 -> sTmIn_D_u8VcEvHiSidePSB/1  "sTmIn_D_u8VcEvHiSidePSB"
  Event_DTC_128D11_GetEventStatus/1 -> InDebug23/1
  InDebug23/1 -> sTmIn_D_u8VcEvHiSideTmpSnrSG/1  "sTmIn_D_u8VcEvHiSideTmpSnrSG"
  Event_DTC_128D15_GetEventStatus/1 -> InDebug24/1
  InDebug24/1 -> sTmIn_D_u8VcEvOutrCondOutTOP/1  "sTmIn_D_u8VcEvOutrCondOutTOP"
  Event_DTC_507011_GetEventStatus/1 -> InDebug25/1
  InDebug25/1 -> sTmIn_D_u8VcEvChillerOutTSG/1  "sTmIn_D_u8VcEvChillerOutTSG"
  Event_DTC_507015_GetEventStatus/1 -> InDebug26/1
  InDebug26/1 -> sTmIn_D_u8VcEvChillerOutTOP/1  "sTmIn_D_u8VcEvChillerOutTOP"
  Event_DTC_507111_GetEventStatus/1 -> InDebug27/1
  InDebug27/1 -> sTmIn_D_u8VcEvInrCondOutTSG/1  "sTmIn_D_u8VcEvInrCondOutTSG"
  Event_DTC_507115_GetEventStatus/1 -> InDebug28/1
  InDebug28/1 -> sTmIn_D_u8VcEvInrCondOutTOP/1  "sTmIn_D_u8VcEvInrCondOutTOP"
  Event_DTC_507C11_GetEventStatus/1 -> InDebug29/1
  InDebug29/1 -> sTmIn_D_u8VcEvEvapOutTSG/1  "sTmIn_D_u8VcEvEvapOutTSG"
  Event_DTC_507C15_GetEventStatus/1 -> InDebug30/1
  InDebug30/1 -> sTmIn_D_u8VcEvEvapOutTOP/1  "sTmIn_D_u8VcEvEvapOutTOP"
  Event_DTC_508C11_GetEventStatus/1 -> InDebug31/1
  InDebug31/1 -> sTmIn_D_u8VcEvCmprDischrgTSG/1  "sTmIn_D_u8VcEvCmprDischrgTSG"
  Event_DTC_508C15_GetEventStatus/1 -> InDebug32/1
  InDebug32/1 -> sTmIn_D_u8VcEvCmprDischrgTOP/1  "sTmIn_D_u8VcEvCmprDischrgTOP"
  Event_DTC_0A0011_GetEventStatus/1 -> InDebug33/1
  InDebug33/1 -> sTmIn_D_u8VcEvTmpClSrSG/1  "sTmIn_D_u8VcEvTmpClSrSG"
  Event_DTC_0A0015_GetEventStatus/1 -> InDebug34/1
  InDebug34/1 -> sTmIn_D_u8VcEvTmpClSrOP/1  "sTmIn_D_u8VcEvTmpClSrOP"
  Event_DTC_131F9C_GetEventStatus/1 -> InDebug35/1
  InDebug35/1 -> sTmIn_D_u8VcEvELDTCooltLvlLo/1  "sTmIn_D_u8VcEvELDTCooltLvlLo"
  Event_DTC_10687A_GetEventStatus/1 -> InDebug36/1
  InDebug36/1 -> sTmIn_D_u8VcEvBattCooltLvlLo/1  "sTmIn_D_u8VcEvBattCooltLvlLo"
  Event_DTC_91FF12_GetEventStatus/1 -> InDebug37/1
  InDebug37/1 -> sTmIn_D_u8VcEvNoHpHighSidePSnrSB/1  "sTmIn_D_u8VcEvNoHpHighSidePSnrSB"
  Event_DTC_91FF14_GetEventStatus/1 -> InDebug38/1
  InDebug38/1 -> sTmIn_D_u8VcEvNoHpHighSidePSnrOP/1  "sTmIn_D_u8VcEvNoHpHighSidePSnrOP"
  yGlAcHpM_B_HpmSov1Actv2FReq/1 -> InDebug39/1
  InDebug39/1 -> yTmIn_B_HpmSov1Actv2FReq/1  "yTmIn_B_HpmSov1Actv2FReq"
  yGlAcHpM_B_HpmSov1ActvCmd2F/1 -> InDebug40/1
  InDebug40/1 -> yTmIn_B_HpmSov1ActvCmd2F/1  "yTmIn_B_HpmSov1ActvCmd2F"
  yGlAcHpM_B_HpmSov2Actv2FReq/1 -> InDebug41/1
  InDebug41/1 -> yTmIn_B_HpmSov2Actv2FReq/1  "yTmIn_B_HpmSov2Actv2FReq"
  yGlAcHpM_B_HpmSov2ActvCmd2F/1 -> InDebug42/1
  InDebug42/1 -> yTmIn_B_HpmSov2ActvCmd2F/1  "yTmIn_B_HpmSov2ActvCmd2F"
  yGlAcHpM_B_HpmSov3Actv2FReq/1 -> InDebug43/1
  InDebug43/1 -> yTmIn_B_HpmSov3Actv2FReq/1  "yTmIn_B_HpmSov3Actv2FReq"
  yGlAcHpM_B_HpmSov3ActvCmd2F/1 -> InDebug44/1
  InDebug44/1 -> yTmIn_B_HpmSov3ActvCmd2F/1  "yTmIn_B_HpmSov3ActvCmd2F"
  yVcEac_B_ChillerValve2FReq/1 -> InDebug45/1
  InDebug45/1 -> yTmIn_B_ChillerValve2FReq/1  "yTmIn_B_ChillerValve2FReq"
  yVcEac_B_ChillerValveReq2F/1 -> InDebug46/1
  InDebug46/1 -> yTmIn_B_ChillerValveReq2F/1  "yTmIn_B_ChillerValveReq2F"
  yVcAc_B_EvaprVlvFrnt2FReq/1 -> InDebug47/1
  InDebug47/1 -> yTmIn_B_EvaprVlvFrnt2FReq/1  "yTmIn_B_EvaprVlvFrnt2FReq"
  yVcAc_B_EvaprVlvReqFrnt2F/1 -> InDebug48/1
  InDebug48/1 -> yTmIn_B_EvaprVlvReqFrnt2F/1  "yTmIn_B_EvaprVlvReqFrnt2F"
  yVcTmAf_B_FanPwm2FReq/1 -> InDebug49/1
  InDebug49/1 -> yTmIn_B_FanPwm2FReq/1  "yTmIn_B_FanPwm2FReq"
  sVcTmAf_X_FanPwmReq2F/1 -> InDebug50/1
  InDebug50/1 -> sTmIn_X_s32FanPwmReq2F/1  "sTmIn_X_s32FanPwmReq2F"
  yGlTmHgMgt_B_PTCPumpSpd2FReq/1 -> InDebug51/1
  InDebug51/1 -> yTmIn_B_PTCPumpSpd2FReq/1  "yTmIn_B_PTCPumpSpd2FReq"
  sGlTmHgMgt_X_PTCPumpSpdReq2F/1 -> InDebug52/1
  InDebug52/1 -> sTmIn_X_s32PTCPumpSpdReq2F/1  "sTmIn_X_s32PTCPumpSpdReq2F"
  yGlHwDrvDiag_B_BattPmp2FReq/1 -> InDebug53/1
  InDebug53/1 -> yTmIn_B_BattPmp2FReq/1  "yTmIn_B_BattPmp2FReq"
  sGlTmBcc_X_BattCooltPmpReq2F/1 -> InDebug54/1
  InDebug54/1 -> sTmIn_X_s32BattCooltPmpReq2F/1  "sTmIn_X_s32BattCooltPmpReq2F"
  yVcTmHcc_B_EmCooltPmp2FReq/1 -> InDebug55/1
  InDebug55/1 -> yTmIn_B_EmCooltPmp2FReq/1  "yTmIn_B_EmCooltPmp2FReq"
  sVcTmHcc_X_EmCooltPmpReq2F/1 -> InDebug56/1
  InDebug56/1 -> sTmIn_X_s32EmCooltPmpReq2F/1  "sTmIn_X_s32EmCooltPmpReq2F"
  yVcBctv_B_VlvPos2FReq/1 -> InDebug57/1
  InDebug57/1 -> yTmIn_B_BctvVlvPos2FReq/1  "yTmIn_B_BctvVlvPos2FReq"
  sVcBctv_X_VlvPosReq2F/1 -> InDebug58/1
  InDebug58/1 -> sTmIn_X_u8BctvVlvPosReq2F/1  "sTmIn_X_u8BctvVlvPosReq2F"
